simulink model "controlFlowFlowchart"  (R2024a)
settings: Solver=FixedStepDiscrete  StartTime=0.0  StopTime=10.0  FixedStep=0.1  RelTol=1e-3  EnableMultiTasking=on
values from neighbouring files (symbols this model uses):
  pageType = 2    [controlFlow.mat]
  user = 1    [controlFlow.mat]
libraries: simulink x1
settings Model: Creator=TUF  LastModifiedBy=TUF
settings SolverCC: AlgebraicLoopSolver=TrustRegion  AutoInsertRateTranBlk=on
settings DataIOCC: LimitDataPoints=on
settings OptimizationCC: LifeSpan=inf
settings DebuggingCC: UnconnectedInputMsg=warning  UnconnectedOutputMsg=warning  UnconnectedLineMsg=warning  AllowSymbolicDim=off  SFUnusedDataAndEventsDiag=none  SFUnexpectedBacktrackingDiag=none  SFInvalidInputDataAccessInChartInitDiag=none  SFNoUnconditionalDefaultTransitionDiag=none  SFTransitionOutsideNaturalParentDiag=none  SFUnreachableExecutionPathDiag=none  SFUndirectedBroadcastEventsDiag=none  SFTransitionActionBeforeConditionDiag=none  SFOutputUsedAsStateInMooreChartDiag=none  SFTemporalDelaySmallerThanSampleTimeDiag=none  SFSelfTransitionDiag=none  SFExecutionAtInitializationDiag=none  ArithmeticOperatorsInVariantConditions=warning
settings ModelReferenceCC: EnableRefExpFcnMdlSchedulingChecks=on
settings SFSimCC: SimUseLocalCustomCode=off  CustomCodeUndefinedFunction=UseInterfaceOnly
settings RTWCC: RTWUseLocalCustomCode=off  GPUComputeCapability=3.5  DLArmComputeVersion=19.05
settings CodeAppCC: StateflowObjectComments=on
settings GRTTargetCC: TargetLangStandard=C89/C90 (ANSI)
settings ConfigComp: CovMetricSettings=dw  CovSaveCumulativeToWorkspaceVar=on  CovSaveSingleToWorkspaceVar=on  CovExternalEMLEnable=off

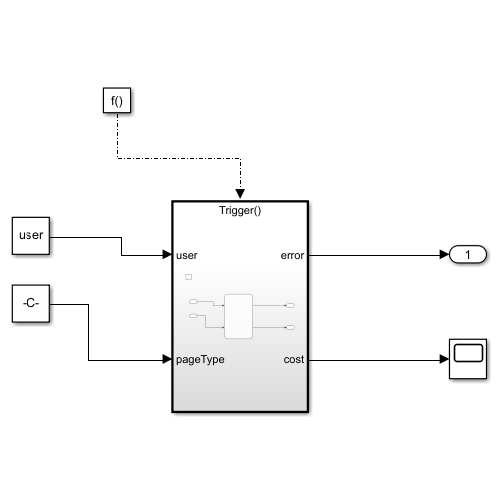
[thumbnail: Simulink's stored preview of the top-level diagram]
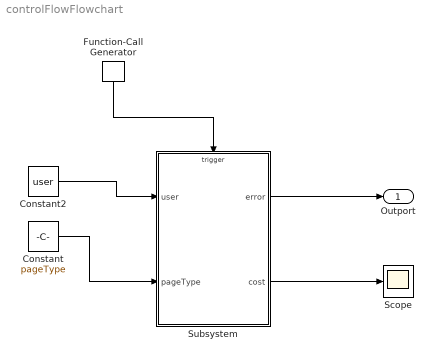
== system controlFlowFlowchart ==
  Constant : Constant  Value=pageType
  Constant2 : Constant  Value=user
  Function-Call Generator : simulink/Ports & Subsystems/Function-Call Generator  sample_time=1  numberOfIterations=1  DisallowWideOutput=off
  Scope : Scope
  Subsystem : Subsystem  TreatAsAtomicUnit=on  SystemSampleTime=1
      settings: MinAlgLoopOccurrences=on
  Outport : Outport
  wires:
  Constant2/1 -> Subsystem/1(user)
  Constant/1 -> Subsystem/2(pageType)
  Subsystem/1(error) -> Outport/1
  Subsystem/2(cost) -> Scope/1
  Function-Call Generator/1 -> Subsystem/Trigger

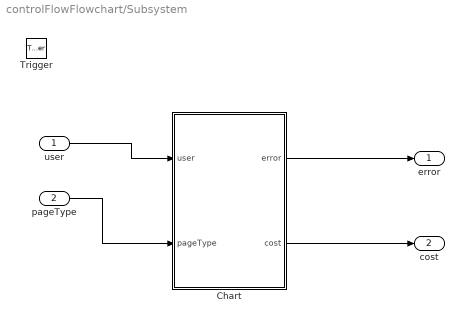
== system controlFlowFlowchart/Subsystem ==
  user : Inport
  pageType : Inport  Port=2
  Trigger : TriggerPort  TriggerType=function-call  VariantControl=(inherit)  PortDimensions=1
  Chart : Stateflow chart  TreatAsAtomicUnit=on
  error : Outport
  cost : Outport  Port=2
  wires:
  user/1 -> Chart/1(user)
  pageType/1 -> Chart/2(pageType)
  Chart/2(cost) -> cost/1
  Chart/1(error) -> error/1

== stateflow chart controlFlowFlowchart/Subsystem/Chart ==
  state initialState
    entry: user == false;
  state sessionBegin
  state cancelSession
  state uploadDocuments
  state choosePageType
  state choosenType1
    rate = 1.5;
  state choosenTypeNull
    rate = 0;
  state choosenType2
    rate = 2;
  state choosenType3
    rate = 3;
  state copies
    copiesPrint = numCopies;
  state colourPrint
    cost = rate*numCopies*2;
  state blackAndWhite
    cost = rate*numCopies*1;
  state displayQR
    display == true;
  state paymentTrue
    printStart = true;
  state paymentFalse
    printStart = false;
  state printDone
  state noPrinting
    error = 1;
  state errorCatch
    error = 0;
  state refunding
    start : error == 0
    refund = true;
  (default) -> initialState
  initialState -> sessionBegin : [user == true]
  sessionBegin -> cancelSession [order 1] : [webPageActive == false]
  cancelSession -> sessionBegin [order 1] : [noActivity == true]
  sessionBegin -> uploadDocuments [order 2] : [webPageActive == true]
  uploadDocuments -> cancelSession [order 2] : [docUpld == false]
  cancelSession -> (junction 87) [order 2]
  paymentFalse -> cancelSession : [paymentDone == false]
  choosenTypeNull -> cancelSession : [pageType == 0]
  uploadDocuments -> choosePageType [order 1] : [docUpld == true]
  choosePageType -> choosenTypeNull [order 4] : [pageType == 0]
  choosePageType -> choosenType1 [order 1] : [pageType == 1]
  choosePageType -> choosenType2 [order 2] : [pageType == 2]
  choosePageType -> choosenType3 [order 3] : [pageType == 3]
  choosenType3 -> copies : [numCopies>0 && rate == 3]
  choosenType2 -> copies : [numCopies > 0 && rate == 2]
  choosenType1 -> copies : [numCopies > 0 && rate == 1.5]
  copies -> blackAndWhite [order 1] : [bw == true]
  copies -> colourPrint [order 2] : [bw == false]
  blackAndWhite -> displayQR : [rate > 0]
  colourPrint -> displayQR : [rate > 0]
  displayQR -> paymentTrue [order 1] : [paymentDone == true]
  displayQR -> paymentFalse [order 2] : [paymentDone == false]
  paymentTrue -> printDone [order 1] : [printComplete == true]
  paymentTrue -> noPrinting [order 2] : [printComplete == false]
  refunding -> errorCatch [order 2] : [refund == false]
  errorCatch -> printDone [order 1] : [error == 0]
  noPrinting -> errorCatch
  errorCatch -> refunding [order 2] : [error == 1]
  printDone -> (junction 74) : [printComplete == true]
  refunding -> (junction 87) [order 1] : [refund == true]
  data: user input; pageType input; start constant double; copiesPrint local; numCopies constant double; bw constant double; error output; cost output; printStart local; refund local; rate local double; noActivity constant double
  events: display local FUNCTION_CALL_EVENT; paymentDone local FUNCTION_CALL_EVENT; printComplete local FUNCTION_CALL_EVENT; webPageActive local RISING_EDGE_EVENT; docUpld local RISING_EDGE_EVENT
